simulink model "NOx_INTEGRATED_REFRANCE_MODEL"  (R2019a)
settings: Solver=VariableStepAuto  StartTime=0.0  StopTime=10.0  RelTol=1e-3
settings Model: Creator=User  LastModifiedBy=User
settings DebuggingCC: SignalInfNanChecking=warning  UniqueDataStoreMsg=warning  StrictBusMsg=ErrorOnBusTreatedAsVector

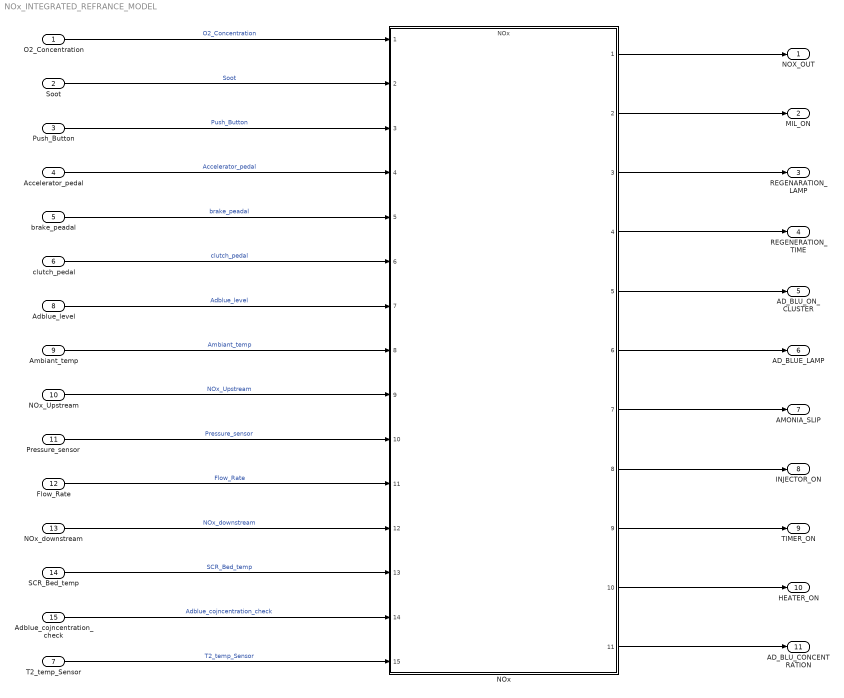
== system NOx_INTEGRATED_REFRANCE_MODEL ==
  O2_Concentration : Inport
  Soot : Inport  Port=2
  Push_Button : Inport  Port=3
  Accelerator_pedal : Inport  Port=4
  brake_peadal : Inport  Port=5
  clutch_pedal : Inport  Port=6
  T2_temp_Sensor : Inport  Port=7
  Adblue_level : Inport  Port=8
  Ambiant_temp : Inport  Port=9
  NOx_Upstream : Inport  Port=10
  Pressure_sensor : Inport  Port=11
  Flow_Rate : Inport  Port=12
  NOx_downstream : Inport  Port=13
  SCR_Bed_temp : Inport  Port=14
  Adblue_cojncentration_check : Inport  Port=15
  NOx : ModelReference  ModelNameDialog=NOx  SimulationMode=Normal  ModelReferenceVersion=1.1
  NOX_OUT : Outport
  MIL_ON : Outport  Port=2
  REGENARATION_LAMP : Outport  Port=3
  REGENERATION_TIME : Outport  Port=4
  AD_BLU_ON_CLUSTER : Outport  Port=5
  AD_BLUE_LAMP : Outport  Port=6
  AMONIA_SLIP : Outport  Port=7
  INJECTOR_ON : Outport  Port=8
  TIMER_ON : Outport  Port=9
  HEATER_ON : Outport  Port=10
  AD_BLU_CONCENTRATION : Outport  Port=11
  wires:
  Ambiant_temp/1 -> NOx/8  "Ambiant_temp"
  NOx/6 -> AD_BLUE_LAMP/1
  NOx/8 -> INJECTOR_ON/1
  NOx/4 -> REGENERATION_TIME/1
  NOx/11 -> AD_BLU_CONCENTRATION/1
  NOx/10 -> HEATER_ON/1
  T2_temp_Sensor/1 -> NOx/15  "T2_temp_Sensor"
  NOx/9 -> TIMER_ON/1
  NOx/7 -> AMONIA_SLIP/1
  Soot/1 -> NOx/2  "Soot"
  Pressure_sensor/1 -> NOx/10  "Pressure_sensor"
  Flow_Rate/1 -> NOx/11  "Flow_Rate"
  SCR_Bed_temp/1 -> NOx/13  "SCR_Bed_temp"
  NOx/2 -> MIL_ON/1
  NOx/3 -> REGENARATION_LAMP/1
  Adblue_level/1 -> NOx/7  "Adblue_level"
  clutch_pedal/1 -> NOx/6  "clutch_pedal"
  NOx/1 -> NOX_OUT/1
  Push_Button/1 -> NOx/3  "Push_Button"
  NOx/5 -> AD_BLU_ON_CLUSTER/1
  Accelerator_pedal/1 -> NOx/4  "Accelerator_pedal"
  Adblue_cojncentration_check/1 -> NOx/14  "Adblue_cojncentration_check"
  NOx_Upstream/1 -> NOx/9  "NOx_Upstream"
  NOx_downstream/1 -> NOx/12  "NOx_downstream"
  O2_Concentration/1 -> NOx/1  "O2_Concentration"
  brake_peadal/1 -> NOx/5  "brake_peadal"
